simulink model "SOP_OL_Harness"  (R2017b)
settings: Solver=FixedStepAuto  StartTime=0.0  StopTime=sim_time  FixedStep=sample_time  RelTol=1e-3  EnableMultiTasking=on
settings Model: Creator=favv5g  LastModifiedBy=nctzv8
settings DataIOCC: LimitDataPoints=on
settings OptimizationCC: LifeSpan=inf
settings DebuggingCC: InheritedTsInSrcMsg=none  AllowSymbolicDim=off  SFUnexpectedBacktrackingDiag=warning  SFNoUnconditionalDefaultTransitionDiag=warning  SFExecutionAtInitializationDiag=none
settings ModelReferenceCC: PropagateSignalLabelsOutOfModel=off
settings CodeAppCC: StateflowObjectComments=on
settings GRTTargetCC: TargetLangStandard=C89/C90 (ANSI)
settings ConfigComp: CovMetricSettings=dw  CovHtmlReporting=on  CovSaveCumulativeToWorkspaceVar=on  CovSaveSingleToWorkspaceVar=on  CovExternalEMLEnable=off

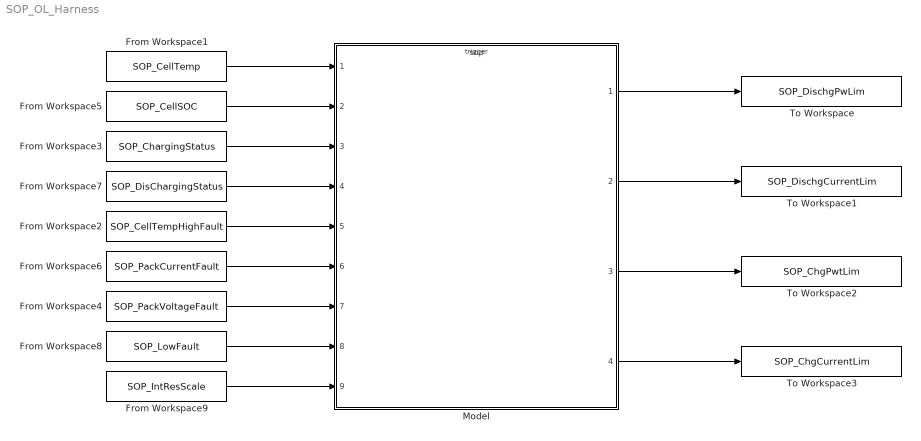
== system SOP_OL_Harness ==
  From Workspace1 : FromWorkspace  VariableName=SOP_CellTemp
  From Workspace2 : FromWorkspace  VariableName=SOP_CellTempHighFault
  From Workspace3 : FromWorkspace  VariableName=SOP_ChargingStatus
  From Workspace4 : FromWorkspace  VariableName=SOP_PackVoltageFault
  From Workspace5 : FromWorkspace  VariableName=SOP_CellSOC
  From Workspace6 : FromWorkspace  VariableName=SOP_PackCurrentFault
  From Workspace7 : FromWorkspace  VariableName=SOP_DisChargingStatus
  From Workspace8 : FromWorkspace  VariableName=SOP_LowFault
  From Workspace9 : FromWorkspace  VariableName=SOP_IntResScale
  Model : ModelReference  ModelNameDialog=sop.slx  SimulationMode=Normal  ModelReferenceVersion=1.50  TriggerPortName=Trigger  TriggerPortTriggerType=function-call  TriggerPortStatesWhenEnabling=held
  To Workspace : ToWorkspace  VariableName=SOP_DischgPwLim  SaveFormat=Timeseries  SampleTime=-1
  To Workspace1 : ToWorkspace  VariableName=SOP_DischgCurrentLim  SaveFormat=Timeseries  SampleTime=-1
  To Workspace2 : ToWorkspace  VariableName=SOP_ChgPwtLim  SaveFormat=Timeseries  SampleTime=-1
  To Workspace3 : ToWorkspace  VariableName=SOP_ChgCurrentLim  SaveFormat=Timeseries  SampleTime=-1
  wires:
  Model/1 -> To Workspace/1
  From Workspace5/1 -> Model/2
  From Workspace1/1 -> Model/1
  From Workspace3/1 -> Model/3
  From Workspace7/1 -> Model/4
  From Workspace2/1 -> Model/5
  From Workspace6/1 -> Model/6
  From Workspace4/1 -> Model/7
  Model/2 -> To Workspace1/1
  Model/3 -> To Workspace2/1
  Model/4 -> To Workspace3/1
  From Workspace8/1 -> Model/8
  From Workspace9/1 -> Model/9
